simulink model "matlab_task"  (R2020a)
settings: Solver=VariableStepAuto  StartTime=0.0  StopTime=10.0  RelTol=1e-3
undefined symbols (not defined in the file): D1, Delta
libraries: powerlib x18, sps_avr x3
settings Model: Creator=Savindu Dilshan  LastModifiedBy=Savindu Dilshan

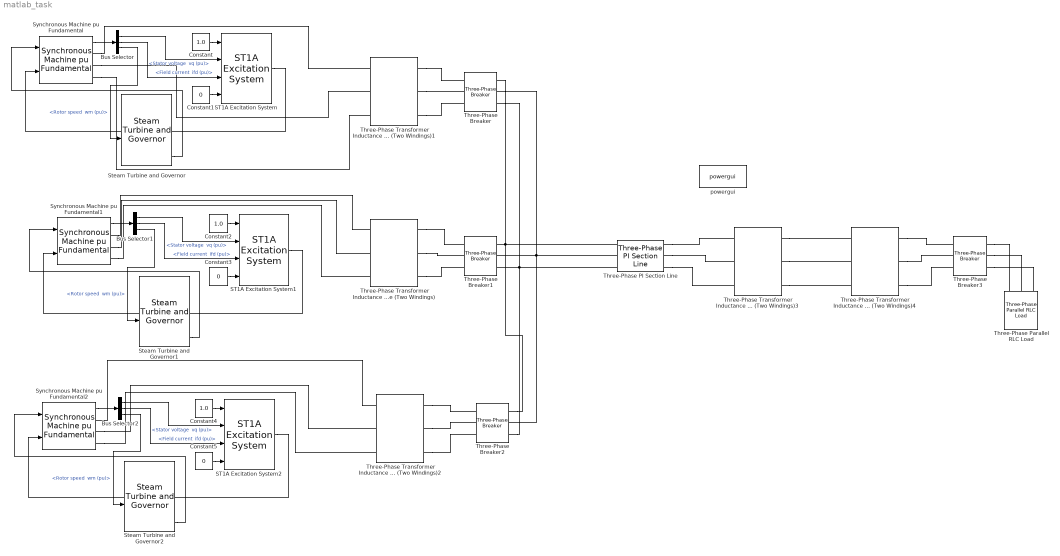
== system matlab_task ==
  Bus Selector : BusSelector  OutputSignals="dq0 components.Stator voltage  vq (pu),dq0 components.Field current  ifd (pu),Mechanical.Rotor speed  wm (pu)"
  Bus Selector1 : BusSelector  OutputSignals="dq0 components.Stator voltage  vq (pu),dq0 components.Field current  ifd (pu),Mechanical.Rotor speed  wm (pu)"
  Bus Selector2 : BusSelector  OutputSignals="dq0 components.Stator voltage  vq (pu),dq0 components.Field current  ifd (pu),Mechanical.Rotor speed  wm (pu)"
  Constant : Constant  Value=1.0
  Constant1 : Constant  Value=0
  Constant2 : Constant  Value=1.0
  Constant3 : Constant  Value=0
  Constant4 : Constant  Value=1.0
  Constant5 : Constant  Value=0
  ST1A Excitation System : sps_avr/ST1A Excitation System  Tr=20e-3  KaTa=[210 0.001]  VIminmax=[-999 +999]  VAminmax=[-999 999]  VRminmax=[-6.0 6.43]  KfTf=[0.001 1]  TbTc=[0 0 0 0]  KLR=1  ILR=2  Kc=0.038  v0=[1 1]  TsBlock=0
      settings: SourceProductBaseCode=PS
  ST1A Excitation System1 : sps_avr/ST1A Excitation System  Tr=20e-3  KaTa=[210 0.001]  VIminmax=[-999 +999]  VAminmax=[-999 999]  VRminmax=[-6.0 6.43]  KfTf=[0.001 1]  TbTc=[0 0 0 0]  KLR=1  ILR=2  Kc=0.038  v0=[1 1]  TsBlock=0
      settings: SourceProductBaseCode=PS
  ST1A Excitation System2 : sps_avr/ST1A Excitation System  Tr=20e-3  KaTa=[210 0.001]  VIminmax=[-999 +999]  VAminmax=[-999 999]  VRminmax=[-6.0 6.43]  KfTf=[0.001 1]  TbTc=[0 0 0 0]  KLR=1  ILR=2  Kc=0.038  v0=[1 1]  TsBlock=0
      settings: SourceProductBaseCode=PS
  Steam Turbine and Governor : powerlib/Machines/Steam Turbine and Governor  gentype=Tandem-compound (multi-mass)  reg1="[ 1  0.05    0 ]"  reg2="[ 0.001  0.15 ]"  reg3="[ -0.1  0.1  0  4.496]"  N=3600  turb1="[ 0  10   3.3   0.5   ]"  turb2="[ 0.5   0.5   0  0 ]"  HA="[  1.5498   0.24894  0  0 ]"  KA="[  83.47  42.702  0  0 ]"  DA="[  0.3104  0.05  0  0 ]*8"  ini1=250.35/555  ini2=[2.7247e-008,-120.13]
      settings: SourceProductBaseCode=PS
  Steam Turbine and Governor1 : powerlib/Machines/Steam Turbine and Governor  gentype=Tandem-compound (multi-mass)  reg1="[ 1  0.05    0 ]"  reg2="[ 0.001  0.15 ]"  reg3="[ -0.1  0.1  0  4.496]"  N=3600  turb1="[ 0  10   3.3   0.5   ]"  turb2="[ 0.5   0.5   0  0 ]"  HA="[  1.5498   0.24894  0  0 ]"  KA="[  83.47  42.702  0  0 ]"  DA="[  0.3104  0.05  0  0 ]*8"  ini1=250.35/555  ini2=[2.7247e-008,-120.13]
      settings: SourceProductBaseCode=PS
  Steam Turbine and Governor2 : powerlib/Machines/Steam Turbine and Governor  gentype=Tandem-compound (multi-mass)  reg1="[ 1  0.05    0 ]"  reg2="[ 0.001  0.15 ]"  reg3="[ -0.1  0.1  0  4.496]"  N=3600  turb1="[ 0  10   3.3   0.5   ]"  turb2="[ 0.5   0.5   0  0 ]"  HA="[  1.5498   0.24894  0  0 ]"  KA="[  83.47  42.702  0  0 ]"  DA="[  0.3104  0.05  0  0 ]*8"  ini1=250.35/555  ini2=[2.7247e-008,-120.13]
      settings: SourceProductBaseCode=PS
  Synchronous Machine pu Fundamental : powerlib/Machines/Synchronous Machine pu Fundamental  PresetModel=No  MechanicalLoad=Mechanical power Pm  ShowDetailedParameters=on  RotorType=Salient-pole  Units=per unit fundamental parameters  MeasurementBus=off  NominalParameters=[1e6 11e3 50]  Stator="[ 2.85E-03  0.114  1.19  0.36 ]"  Field="[ 5.79E-04  0.114]"  Dampers2=[0.0652, 0.5134, 0.0287, 0.2553, 7.765e-3, 0.9167 ]  Dampers1="[ 1.17E-02  0.182  1.97E-02  0.384 ]"  Mechanical=[ 3.7 0 20]  PolePairs=20  InitialConditions="[ 0  0  0  0  0  0  0  0  1 ]"  SetSaturation=off  Saturation=[0.6404,0.7127,0.8441,0.9214,0.9956,1.082,1.19,1.316,1.457;0.7,0.7698,0.8872,0.9466,0.9969,1.046,1.1,1.151,1.201]  LoadFlowParameters=[1,0,0,0,0]  TsPowergui=0  TsBlock=-1  IterativeModel=Trapezoidal non iterative  IterativeDiscreteModel=Trapezoidal non iterative  BusType=PV  Pref=1e6  Qref=0  Qmin=-inf  Qmax=inf  PLF=0  QLF=0
      settings: SourceProductBaseCode=PS
  Synchronous Machine pu Fundamental1 : powerlib/Machines/Synchronous Machine pu Fundamental  PresetModel=No  MechanicalLoad=Mechanical power Pm  ShowDetailedParameters=on  RotorType=Salient-pole  Units=per unit fundamental parameters  MeasurementBus=off  NominalParameters=[2e6 12e3 50]  Stator="[ 2.85E-03  0.114  1.19  0.36 ]"  Field="[ 5.79E-04  0.114]"  Dampers2=[0.0652, 0.5134, 0.0287, 0.2553, 7.765e-3, 0.9167 ]  Dampers1="[ 1.17E-02  0.182  1.97E-02  0.384 ]"  Mechanical=[ 3.7 0 20]  PolePairs=20  InitialConditions="[ 0  0  0  0  0  0  0  0  1 ]"  SetSaturation=off  Saturation=[0.6404,0.7127,0.8441,0.9214,0.9956,1.082,1.19,1.316,1.457;0.7,0.7698,0.8872,0.9466,0.9969,1.046,1.1,1.151,1.201]  LoadFlowParameters=[1,0,0,0,0]  TsPowergui=0  TsBlock=-1  IterativeModel=Trapezoidal non iterative  IterativeDiscreteModel=Trapezoidal non iterative  BusType=PV  Pref=2e6  Qref=0  Qmin=-inf  Qmax=inf  PLF=0  QLF=0
      settings: SourceProductBaseCode=PS
  Synchronous Machine pu Fundamental2 : powerlib/Machines/Synchronous Machine pu Fundamental  PresetModel=No  MechanicalLoad=Mechanical power Pm  ShowDetailedParameters=on  RotorType=Salient-pole  Units=per unit fundamental parameters  MeasurementBus=off  NominalParameters=[4e6 10e3 50]  Stator="[ 2.85E-03  0.114  1.19  0.36 ]"  Field="[ 5.79E-04  0.114]"  Dampers2=[0.0652, 0.5134, 0.0287, 0.2553, 7.765e-3, 0.9167 ]  Dampers1="[ 1.17E-02  0.182  1.97E-02  0.384 ]"  Mechanical=[ 3.7 0 20]  PolePairs=20  InitialConditions="[ 0  0  0  0  0  0  0  0  1 ]"  SetSaturation=off  Saturation=[0.6404,0.7127,0.8441,0.9214,0.9956,1.082,1.19,1.316,1.457;0.7,0.7698,0.8872,0.9466,0.9969,1.046,1.1,1.151,1.201]  LoadFlowParameters=[1,0,0,0,0]  TsPowergui=0  TsBlock=-1  IterativeModel=Trapezoidal non iterative  IterativeDiscreteModel=Trapezoidal non iterative  BusType=PV  Pref=4e6  Qref=0  Qmin=-inf  Qmax=inf  PLF=0  QLF=0
      settings: SourceProductBaseCode=PS
  Three-Phase PI Section Line : powerlib/Elements/Three-Phase PI Section Line  LConnTagsString=a|b|c  RConnTagsString=A|B|C  Frequency=60  Resistances=[ 0.01273 0.3864]  Inductances="[ 0.9337e-3  4.1264e-3]"  Capacitances=[12.74e-9 7.751e-9]  Length=100
  Three-Phase Parallel RLC Load : powerlib/Elements/Three-Phase Parallel RLC Load  LConnTagsString=A|B|C  Configuration=Y (grounded)  NominalVoltage=400  Vabc=[230 230 230]  Vabcp=[1e3 1e3 1e3]  NominalFrequency=50  UnbalancedPower=on  ActivePower=10e3  InductivePower=100  CapacitivePower=100  Pabc=[666667 666667 666667]  QLabc=[0 0 0]  QCabc=[0 0 0]  Pabcp=[10e3 9e3 11e3]  QLabcp=[100 90 110]  QCabcp=[100 90 110]  Measurements=None  LoadType=constant Z
  Three-Phase Breaker{,1..3} (4 alike) : powerlib/Elements/Three-Phase Breaker  InitialState=open  SwitchA=on  SwitchB=on  SwitchC=on  SwitchTimes="[1/60  5/60]"  External=off  BreakerResistance=0.01  SnubberResistance=1e6  SnubberCapacitance=inf  Measurements=None
  Three-Phase Transformer Inductance Matrix Type (Two Windings) : powerlib/Elements/Three-Phase Transformer Inductance Matrix Type (Two Windings)  CoreType=Three-limb or five-limb core  Winding1Connection=Delta (D1)  Winding2Connection=Yg  AutoTransformer=off  Measurements=None  NominalPower=[2.5e6, 50]  VLLnom=[12e3, 132e3]  WindingResistances=[0.008, 0.008]  NoLoadIexcPos=1.5  NoLoadPlossPos=2000  ShortCircuitReactancePos=0.08  ShortCircuitReactancePosAuto=0.06  NoLoadIexcZero=100  NoLoadPlossZero=1500  ShortCircuitReactanceZero=0.03  ShortCircuitReactanceZeroAuto=0.03
      settings: SourceProductBaseCode=PS
  Three-Phase Transformer Inductance Matrix Type (Two Windings)1 : powerlib/Elements/Three-Phase Transformer Inductance Matrix Type (Two Windings)  CoreType=Three-limb or five-limb core  Winding1Connection=Delta (D1)  Winding2Connection=Yg  AutoTransformer=off  Measurements=None  NominalPower=[1.25e6, 50]  VLLnom=[11e3, 132e3]  WindingResistances=[0.008, 0.008]  NoLoadIexcPos=1.5  NoLoadPlossPos=1500  ShortCircuitReactancePos=0.08  ShortCircuitReactancePosAuto=0.06  NoLoadIexcZero=100  NoLoadPlossZero=1500  ShortCircuitReactanceZero=0.03  ShortCircuitReactanceZeroAuto=0.03
      settings: SourceProductBaseCode=PS
  Three-Phase Transformer Inductance Matrix Type (Two Windings)2 : powerlib/Elements/Three-Phase Transformer Inductance Matrix Type (Two Windings)  CoreType=Three-limb or five-limb core  Winding1Connection=Delta (D1)  Winding2Connection=Yg  AutoTransformer=off  Measurements=None  NominalPower=[5e6, 50]  VLLnom=[10e3, 132e3]  WindingResistances=[0.007, 0.007]  NoLoadIexcPos=1.5  NoLoadPlossPos=3000  ShortCircuitReactancePos=0.09  ShortCircuitReactancePosAuto=0.06  NoLoadIexcZero=100  NoLoadPlossZero=1500  ShortCircuitReactanceZero=0.03  ShortCircuitReactanceZeroAuto=0.03
      settings: SourceProductBaseCode=PS
  Three-Phase Transformer Inductance Matrix Type (Two Windings)3 : powerlib/Elements/Three-Phase Transformer Inductance Matrix Type (Two Windings)  CoreType=Three-limb or five-limb core  Winding1Connection=Yg  Winding2Connection=Yg  AutoTransformer=off  Measurements=None  NominalPower=[10e6, 50]  VLLnom=[132e3, 11e3]  WindingResistances=[0.008, 0.008]  NoLoadIexcPos=1  NoLoadPlossPos=4000  ShortCircuitReactancePos=0.10  ShortCircuitReactancePosAuto=0.06  NoLoadIexcZero=100  NoLoadPlossZero=1500  ShortCircuitReactanceZero=0.03  ShortCircuitReactanceZeroAuto=0.03
      settings: SourceProductBaseCode=PS
  Three-Phase Transformer Inductance Matrix Type (Two Windings)4 : powerlib/Elements/Three-Phase Transformer Inductance Matrix Type (Two Windings)  CoreType=Three-limb or five-limb core  Winding1Connection=Delta (D1)  Winding2Connection=Yg  AutoTransformer=off  Measurements=None  NominalPower=[10e6, 50]  VLLnom=[11e3, 400]  WindingResistances=[0.005 0.005]  NoLoadIexcPos=2  NoLoadPlossPos=3000  ShortCircuitReactancePos=0.06  ShortCircuitReactancePosAuto=0.06  NoLoadIexcZero=100  NoLoadPlossZero=1500  ShortCircuitReactanceZero=0.03  ShortCircuitReactanceZeroAuto=0.03
      settings: SourceProductBaseCode=PS
  powergui : powerlib/powergui  Priority=1  SimulationMode=Continuous  SampleTime=50e-6  frequency=60  Iterations=50  frequencyindice=60  Pbase=100e6  ErrMax=1e-4  UnitsV=kV  UnitsW=MW  buscounter=0  FunctionMessages=off  echomessages=off  EnableUseOfTLC=off  CurrentSourceSwitches=off  DisableSnubberDevices=off  DisableRonSwitches=off  DisableVfSwitches=off  DisplayEquations=off  AutomaticDiscreteSolvers=off  SolverType=Tustin/Backward Euler (TBE)  Interpol=off  ExternalGateDelay=off  methode=off  Ts=100  x0status=blocks  SPID=on  SwTol=0  HookPort=off  NonlinearTolerance=1e-4  nMaxIteration=100  ContinueOnMaxIteration=off  RestoreLinks=warning  ResistiveCurrentMeasurement=off  Frange=[0:2:500]  Ylog=off  Xlog=on  ShowGrid=off  save=off  variable=ZData  structure=0  ZoomFFT=off  StartTime=0.0  cycles=1  DisplayStyle=1  fundamental=60  FreqAxis=off  MaxFrequency=1000  frequencyindicesteady=1  RmsSteady=1  display=off
  wires:
  Synchronous Machine pu Fundamental/1 -> Bus Selector/1
  Bus Selector/1 -> ST1A Excitation System/2  "<Stator voltage  vq (pu)>"
  Bus Selector/2 -> ST1A Excitation System/3  "<Field current  ifd (pu)>"
  ST1A Excitation System/1 -> Synchronous Machine pu Fundamental/2
  Constant/1 -> ST1A Excitation System/1
  Constant1/1 -> ST1A Excitation System/4
  Bus Selector/3 -> Steam Turbine and Governor/3  "<Rotor speed  wm (pu)>"
  Steam Turbine and Governor/4 -> Synchronous Machine pu Fundamental/1
  Bus Selector1/3 -> Steam Turbine and Governor1/3  "<Rotor speed  wm (pu)>"
  Bus Selector1/1 -> ST1A Excitation System1/2  "<Stator voltage  vq (pu)>"
  Bus Selector1/2 -> ST1A Excitation System1/3  "<Field current  ifd (pu)>"
  Synchronous Machine pu Fundamental1/1 -> Bus Selector1/1
  ST1A Excitation System1/1 -> Synchronous Machine pu Fundamental1/2
  Steam Turbine and Governor1/4 -> Synchronous Machine pu Fundamental1/1
  Constant2/1 -> ST1A Excitation System1/1
  Constant3/1 -> ST1A Excitation System1/4
  Bus Selector2/3 -> Steam Turbine and Governor2/3  "<Rotor speed  wm (pu)>"
  Bus Selector2/1 -> ST1A Excitation System2/2  "<Stator voltage  vq (pu)>"
  Bus Selector2/2 -> ST1A Excitation System2/3  "<Field current  ifd (pu)>"
  Synchronous Machine pu Fundamental2/1 -> Bus Selector2/1
  ST1A Excitation System2/1 -> Synchronous Machine pu Fundamental2/2
  Steam Turbine and Governor2/4 -> Synchronous Machine pu Fundamental2/1
  Constant4/1 -> ST1A Excitation System2/1
  Constant5/1 -> ST1A Excitation System2/4
  connections:
  Synchronous Machine pu Fundamental/RConn1 -- Three-Phase Transformer Inductance Matrix Type (Two Windings)1/LConn1
  Synchronous Machine pu Fundamental/RConn2 -- Three-Phase Transformer Inductance Matrix Type (Two Windings)1/LConn2
  Synchronous Machine pu Fundamental/RConn3 -- Three-Phase Transformer Inductance Matrix Type (Two Windings)1/LConn3
  Synchronous Machine pu Fundamental1/RConn1 -- Three-Phase Transformer Inductance Matrix Type (Two Windings)/LConn1
  Synchronous Machine pu Fundamental1/RConn2 -- Three-Phase Transformer Inductance Matrix Type (Two Windings)/LConn2
  Synchronous Machine pu Fundamental1/RConn3 -- Three-Phase Transformer Inductance Matrix Type (Two Windings)/LConn3
  Synchronous Machine pu Fundamental2/RConn1 -- Three-Phase Transformer Inductance Matrix Type (Two Windings)2/LConn1
  Synchronous Machine pu Fundamental2/RConn2 -- Three-Phase Transformer Inductance Matrix Type (Two Windings)2/LConn2
  Synchronous Machine pu Fundamental2/RConn3 -- Three-Phase Transformer Inductance Matrix Type (Two Windings)2/LConn3
  Three-Phase Transformer Inductance Matrix Type (Two Windings)2/RConn1 -- Three-Phase Breaker2/LConn1
  Three-Phase Transformer Inductance Matrix Type (Two Windings)2/RConn2 -- Three-Phase Breaker2/LConn2
  Three-Phase Transformer Inductance Matrix Type (Two Windings)2/RConn3 -- Three-Phase Breaker2/LConn3
  Three-Phase Transformer Inductance Matrix Type (Two Windings)/RConn1 -- Three-Phase Breaker1/LConn1
  Three-Phase Transformer Inductance Matrix Type (Two Windings)/RConn2 -- Three-Phase Breaker1/LConn2
  Three-Phase Transformer Inductance Matrix Type (Two Windings)/RConn3 -- Three-Phase Breaker1/LConn3
  Three-Phase Transformer Inductance Matrix Type (Two Windings)1/RConn1 -- Three-Phase Breaker/LConn1
  Three-Phase Transformer Inductance Matrix Type (Two Windings)1/RConn2 -- Three-Phase Breaker/LConn2
  Three-Phase Transformer Inductance Matrix Type (Two Windings)1/RConn3 -- Three-Phase Breaker/LConn3
  Three-Phase Breaker/RConn1 -- Three-Phase Breaker1/RConn1 -- Three-Phase PI Section Line/LConn1 -- Three-Phase Breaker2/RConn1
  Three-Phase Breaker1/RConn2 -- Three-Phase Breaker2/RConn2 -- Three-Phase PI Section Line/LConn2 -- Three-Phase Breaker/RConn2
  Three-Phase Breaker/RConn3 -- Three-Phase PI Section Line/LConn3 -- Three-Phase Breaker2/RConn3 -- Three-Phase Breaker1/RConn3
  Three-Phase PI Section Line/RConn1 -- Three-Phase Transformer Inductance Matrix Type (Two Windings)3/LConn1
  Three-Phase PI Section Line/RConn2 -- Three-Phase Transformer Inductance Matrix Type (Two Windings)3/LConn2
  Three-Phase PI Section Line/RConn3 -- Three-Phase Transformer Inductance Matrix Type (Two Windings)3/LConn3
  Three-Phase Transformer Inductance Matrix Type (Two Windings)3/RConn1 -- Three-Phase Transformer Inductance Matrix Type (Two Windings)4/LConn1
  Three-Phase Transformer Inductance Matrix Type (Two Windings)3/RConn2 -- Three-Phase Transformer Inductance Matrix Type (Two Windings)4/LConn2
  Three-Phase Transformer Inductance Matrix Type (Two Windings)3/RConn3 -- Three-Phase Transformer Inductance Matrix Type (Two Windings)4/LConn3
  Three-Phase Transformer Inductance Matrix Type (Two Windings)4/RConn1 -- Three-Phase Breaker3/LConn1
  Three-Phase Transformer Inductance Matrix Type (Two Windings)4/RConn2 -- Three-Phase Breaker3/LConn2
  Three-Phase Transformer Inductance Matrix Type (Two Windings)4/RConn3 -- Three-Phase Breaker3/LConn3
  Three-Phase Breaker3/RConn1 -- Three-Phase Parallel RLC Load/LConn1
  Three-Phase Breaker3/RConn2 -- Three-Phase Parallel RLC Load/LConn2
  Three-Phase Breaker3/RConn3 -- Three-Phase Parallel RLC Load/LConn3
